simulink model "ver1_3DOF_draft2"  (R2023b)
settings: Solver=FixedStepAuto  StartTime=5  StopTime=45  RelTol=1e-3
values from neighbouring files (symbols this model uses):
  current_height = 0.0    (= 0)    [wrapper_for_simulink.m]
  current_pitch = 0.0    (= 0)    [wrapper_for_simulink.m]
  current_vel = 0.0    (= 0)    [wrapper_for_simulink.m]
  extension_length = 0.0    (= 0)    [wrapper_for_simulink.m]
undefined symbols (not defined in the file or in its folder): HDBK, Light, magnitude, MIL
libraries: aerolibwind2 x3, aerolibasang x2, aerolibadyn x1, aerolibatmos2 x1
settings Model: Creator=User  LastModifiedBy=User
settings DataIOCC: ReturnWorkspaceOutputsName=tp3ca22a37_fc90_43f8_8ebe_8c0e39ad763e
settings DebuggingCC: AlgebraicLoopMsg=none  ArtificialAlgebraicLoopMsg=none  ModelReferenceExtraNoncontSigs=none  OperatingPointInterfaceChecksumMismatchMsg=none

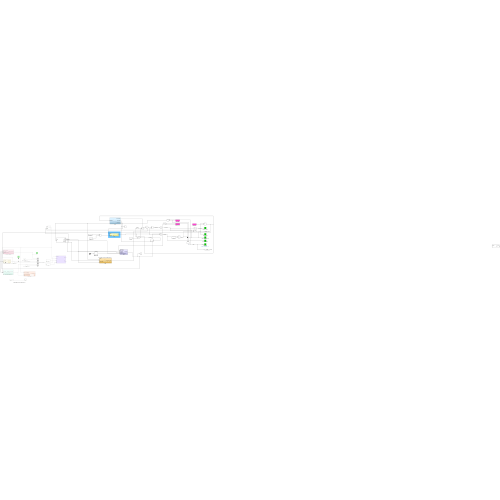
[thumbnail: Simulink's stored preview of the top-level diagram]
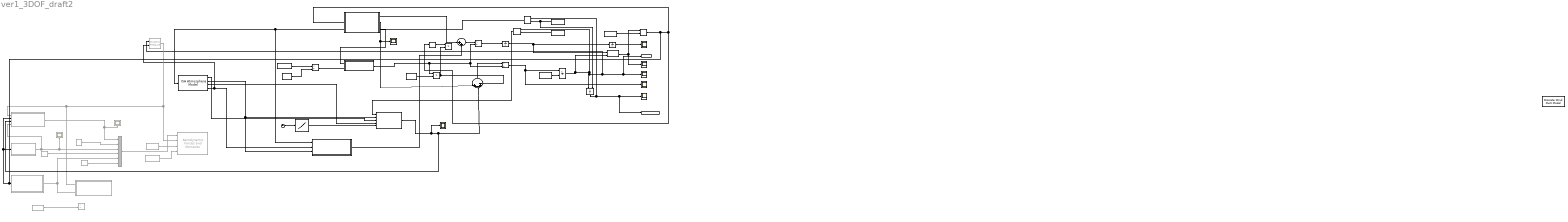
== system ver1_3DOF_draft2 ==
  note: ignore everything after v = 0
  note: need to figure out how the wind parameters here
  note: pitch damping moment: see pg 44 of OR doc
  " m(t)" : Subsystem
  "Aerodynamic Forces and Moments " : aerolibadyn/Aerodynamic Forces and Moments   Commented=on  inputAxes=Body  outputForceAxes=Body  outputMomentAxes=Body  S=0.016513  b=2.91  cbar=0.145
  Atan2 : Trigonometry  Operator=atan2
  Axial force coefficient : Subsystem  Commented=on
  CG rocket : Constant  Commented=on  Value=[0 0 1.16]  VectorParams1D=off
  CP rocket : Constant  Commented=on  Value=[0 0 0.95]  VectorParams1D=off
  Clock : Clock
  Delay1 : Delay  DelayLength=1  InitialConditionSource=Input port
      settings: InputPortMap=u0,p4
  Delay2 : Delay  DelayLength=1  InitialConditionSource=Input port
      settings: InputPortMap=u0,p4
  Delay3 : Delay  DelayLength=1  InitialConditionSource=Input port
      settings: InputPortMap=u0,p4
  Discrete Wind Gust Model : aerolibwind2/Discrete Wind Gust Model  units=Metric (MKS)  Gx=on  Gy=on  Gz=on  t_0=5  d_m=[120 120 80]  v_m=[3.5 3.5 3.0]
  Divide : Product  Inputs=*/
  Divide1 : Product  Inputs=*/
  Divide2 : Product  Inputs=*/
  Divide3 : Product  Commented=on  Inputs=*/
  Dynamic Pressure : aerolibasang/Dynamic Pressure  Commented=on
  Extension Plan : Lookup_n-D  NumberOfTableDimensions=1  BreakpointsForDimension1=[0 4.99 5 5.1 5.11 6]  Table=[0 0 extension_length 0.01*extension_length 0 0]  InternalRulePriority=Speed  RndMeth=Simplest
  Flight path angle : Scope
  ISA Atmosphere Model : aerolibatmos2/ISA Atmosphere Model  useExtended=off  action=Warning  custom=on  viscosityOut=off  g=9.80665  gamma=1.4  R=287.0531  L=0.0065  h_trop=11000  h_strat=20000  rho0=1.002  P0=86503.88  T0=temperature  h0=1401
  Integrator : Integrator  InitialConditionSource=external
  Integrator1 : Integrator  InitialConditionSource=external
  Integrator2 : Integrator
  Integrator3 : Integrator
  Normal Force coefficient : Subsystem  Commented=on
  Pitch moment : Subsystem  Commented=on
  Pitch moment coefficient : Subsystem  Commented=on
  Product1 : Product
  Product2 : Product
  Scope : Scope
  Scope1 : Scope  Commented=on
  Scope2 : Scope
  Scope4 : Scope  Commented=on
  Side force coefficient : Constant  Commented=on  Value=0
  Sin : Trigonometry
  Sum : Sum  Inputs=|+--+-
  Sum1 : Sum  Inputs=|++
  Vector Concatenate : Concatenate  Commented=on  NumInputs=6
  WIND : Subsystem
  current height : Constant  Value=current_height
  current pitch : Constant  Value=current_pitch
  current vel : Constant  Value=current_vel
  current velocity : Constant  Value=current_vel
  drag : Subsystem
  gravity g : Constant  Value=9.80665
  horizontal distance : Scope
  moi : Constant  Commented=on  Value=18.065
  propellant mass : Constant  Value=10.048
  roll moment coefficient : Constant  Commented=on  Value=0
  thrust : Subsystem
  total impulse : Constant  Value=21384.0
  vertical acceleration : Scope
  vertical height : Scope
  vertical velocity in earth ref : Scope
  yaw moment coefficient : Constant  Commented=on  Value=0
  Out1 : Outport  SignalName=height
  Out2 : Outport  Port=2  SignalName=velocity
  wires:
  Integrator1/1 -> Atan2/2, Integrator/1, Dynamic Pressure/1, Out2/1, vertical velocity in earth ref/1, Delay2/1  "velocity"
  ISA Atmosphere Model/2 -> WIND/3(speed of sound), drag/2(speed of sound)  "speed of sound"
  Sum/1 -> Divide1/1
  thrust/2(vertical thrust) -> Scope/1, Sum/1
  Delay2/1 -> drag/1(velocity vector)
  current velocity/1 -> Delay2/2
  current pitch/1 -> Delay1/2
  ISA Atmosphere Model/4 -> Dynamic Pressure/2, WIND/2(In2)
  " m(t)"/1(m(t)) -> Product1/1, Divide1/2, Divide2/2
  thrust/3(magnitude of T) -> " m(t)"/1(thrust)
  Integrator/1 -> Delay3/1, Out1/1, vertical height/1  "height"
  gravity g/1 -> Product1/2
  total impulse/1 -> Divide/1
  propellant mass/1 -> Divide/2
  Divide/1 -> " m(t)"/2(exhaust velocity)
  Divide1/1 -> Integrator1/1, vertical acceleration/1  "vertical accel"
  Atan2/1 -> Delay1/1, Flight path angle/1
  Delay3/1 -> ISA Atmosphere Model/1, WIND/1(Altitude)
  Sum1/1 -> Divide2/1  "Fx"
  WIND/1(wind force u direction) -> Sum1/2
  Integrator2/1 -> Atan2/1, Integrator3/1  "horizontal vel"
  Divide2/1 -> Integrator2/1  "horizontal accel"
  Product1/1 -> Sum/5, Product2/2  "gravitational"
  Sin/1 -> Product2/1
  thrust/1(horizontal thrust) -> Sum1/1
  Clock/1 -> Extension Plan/1
  current vel/1 -> Integrator1/2
  current height/1 -> Delay3/2, Integrator/2
  ISA Atmosphere Model/3 -> drag/4(pressure(Pa))
  Extension Plan/1 -> drag/5(Airbrakes extension plan)
  CG rocket/1 -> "Aerodynamic Forces and Moments "/3
  Vector Concatenate/1 -> "Aerodynamic Forces and Moments "/1  "aerodynamic coefficients"
  yaw moment coefficient/1 -> Vector Concatenate/6
  Pitch moment coefficient/1(pitch moment coefficient) -> Pitch moment/2(pitch moment coefficient), Vector Concatenate/5
  Normal Force coefficient/1(Normal) -> Axial force coefficient/4(Normal Force coefficient), Vector Concatenate/3, Scope1/1  "Normal Force coefficient"
  moi/1 -> Divide3/2
  Side force coefficient/1 -> Vector Concatenate/2
  Dynamic Pressure/1 -> "Aerodynamic Forces and Moments "/2, Pitch moment/1(dynammic pressure), Axial force coefficient/1(dynammic pressure)
  Delay1/1 -> Axial force coefficient/2(pitch angle), Normal Force coefficient/1(pitch angle), Pitch moment coefficient/1(pitch angle), Sin/1, thrust/1(pitch angle)
  CP rocket/1 -> "Aerodynamic Forces and Moments "/4
  Axial force coefficient/1("axial force coefficient ") -> Scope4/1, Vector Concatenate/1
  drag/1(Drag Force) -> Scope2/1, Axial force coefficient/3(Drag Force), Sum/3
  roll moment coefficient/1 -> Vector Concatenate/4
  Integrator3/1 -> horizontal distance/1  "horizontal dist"
  ISA Atmosphere Model/1 -> drag/3(temperature)

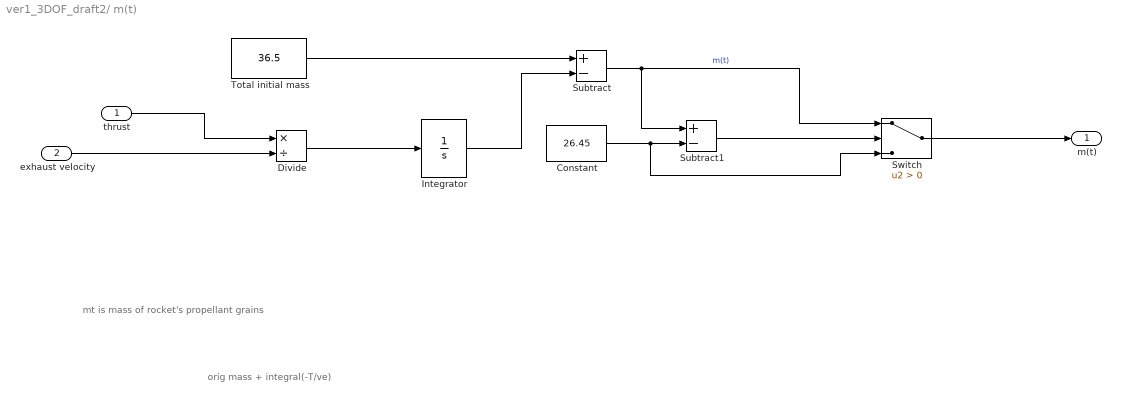
== system ver1_3DOF_draft2/ m(t) ==
  note: orig mass + integral(-T/ve)
  note: mt is mass of rocket's propellant grains
  thrust : Inport
  exhaust velocity : Inport  Port=2
  Constant : Constant  Value=26.45
  Divide : Product  Inputs=*/
  Integrator : Integrator
  Subtract : Sum  Inputs=+-
  Subtract1 : Sum  Inputs=+-
  Switch : Switch  Criteria=u2 > Threshold  SaturateOnIntegerOverflow=off  InputSameDT=off
  Total initial mass : Constant  Value=36.5
  m(t) : Outport
  wires:
  Total initial mass/1 -> Subtract/1
  Subtract/1 -> Subtract1/1, Switch/1  "m(t)"
  thrust/1 -> Divide/1
  exhaust velocity/1 -> Divide/2
  Divide/1 -> Integrator/1
  Integrator/1 -> Subtract/2
  Switch/1 -> m(t)/1
  Constant/1 -> Switch/3, Subtract1/2
  Subtract1/1 -> Switch/2

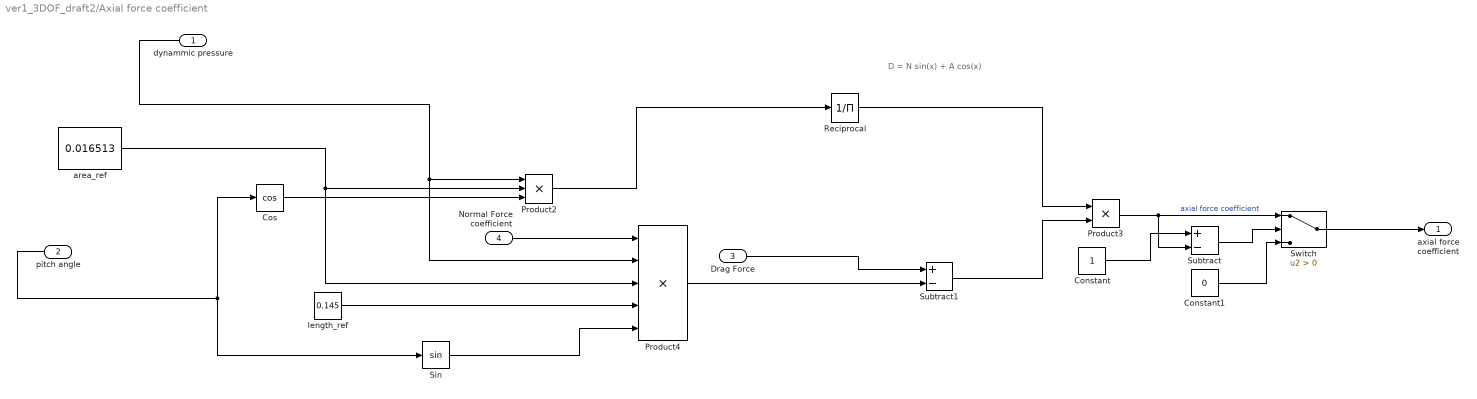
== system ver1_3DOF_draft2/Axial force coefficient ==
  note: D = N sin(x) + A cos(x)
  dynammic pressure : Inport
  pitch angle : Inport  Port=2
  Drag Force : Inport  Port=3
  Normal Force coefficient : Inport  Port=4
  Constant : Constant
  Constant1 : Constant  Value=0
  Cos : Trigonometry  Operator=cos
  Product2 : Product  Inputs=3
  Product3 : Product
  Product4 : Product  Inputs=5
  Reciprocal : Product  Inputs=/
  Sin : Trigonometry
  Subtract : Sum  Inputs=+-
  Subtract1 : Sum  Inputs=+-
  Switch : Switch  Criteria=u2 > Threshold  SaturateOnIntegerOverflow=off  InputSameDT=off
  area_ref : Constant  Value=0.016513
  length_ref : Constant  Value=0.145
  "axial force coefficient " : Outport
  wires:
  Sin/1 -> Product4/5
  pitch angle/1 -> Sin/1, Cos/1
  Normal Force coefficient/1 -> Product4/1
  dynammic pressure/1 -> Product4/2, Product2/1
  area_ref/1 -> Product2/2, Product4/3
  Cos/1 -> Product2/3
  length_ref/1 -> Product4/4
  Product4/1 -> Subtract1/2
  Product3/1 -> Subtract/2, Switch/1  "axial force coefficient"
  Subtract1/1 -> Product3/2
  Drag Force/1 -> Subtract1/1
  Product2/1 -> Reciprocal/1
  Reciprocal/1 -> Product3/1
  Switch/1 -> "axial force coefficient "/1
  Constant/1 -> Subtract/1
  Subtract/1 -> Switch/2
  Constant1/1 -> Switch/3

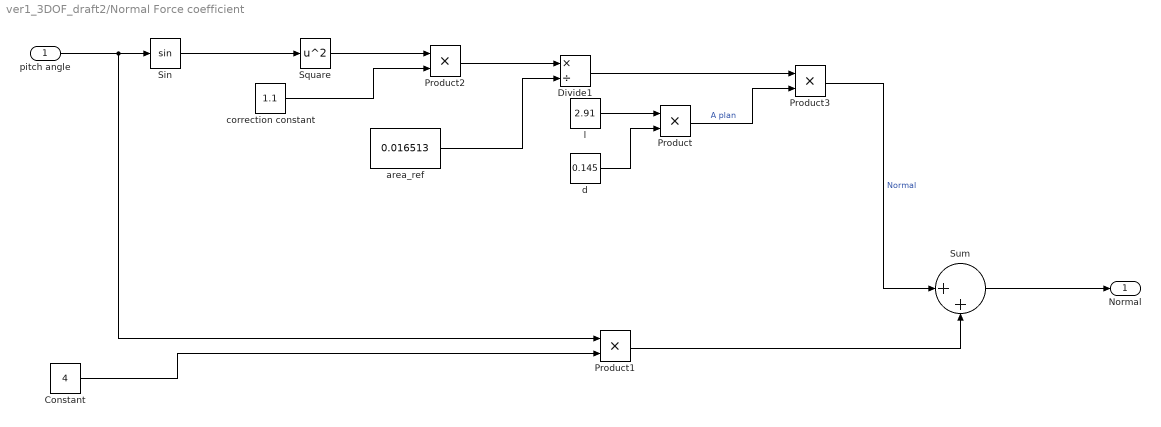
== system ver1_3DOF_draft2/Normal Force coefficient ==
  pitch angle : Inport
  Constant : Constant  Value=4
  Divide1 : Product  Inputs=*/
  Product{,1..3} (4 alike) : Product
  Sin : Trigonometry
  Square : Math  Operator=square
  Sum : Sum  Inputs=|++
  area_ref : Constant  Value=0.016513
  correction constant : Constant  Value=1.1
  d : Constant  Value=0.145
  l : Constant  Value=2.91
  Normal : Outport
  wires:
  pitch angle/1 -> Product1/1, Sin/1
  correction constant/1 -> Product2/2
  Product2/1 -> Divide1/1
  area_ref/1 -> Divide1/2
  Divide1/1 -> Product3/1
  Sin/1 -> Square/1
  Square/1 -> Product2/1
  Product/1 -> Product3/2  "A plan"
  l/1 -> Product/1
  d/1 -> Product/2
  Constant/1 -> Product1/2
  Product1/1 -> Sum/2
  Product3/1 -> Sum/1  "Normal"
  Sum/1 -> Normal/1

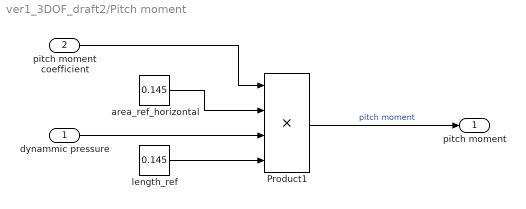
== system ver1_3DOF_draft2/Pitch moment ==
  dynammic pressure : Inport
  pitch moment coefficient : Inport  Port=2
  Product1 : Product  Inputs=4
  area_ref_horizontal : Constant  Value=0.145
  length_ref : Constant  Value=0.145
  pitch moment : Outport
  wires:
  area_ref_horizontal/1 -> Product1/2
  Product1/1 -> pitch moment/1  "pitch moment"
  length_ref/1 -> Product1/4
  dynammic pressure/1 -> Product1/3
  pitch moment coefficient/1 -> Product1/1

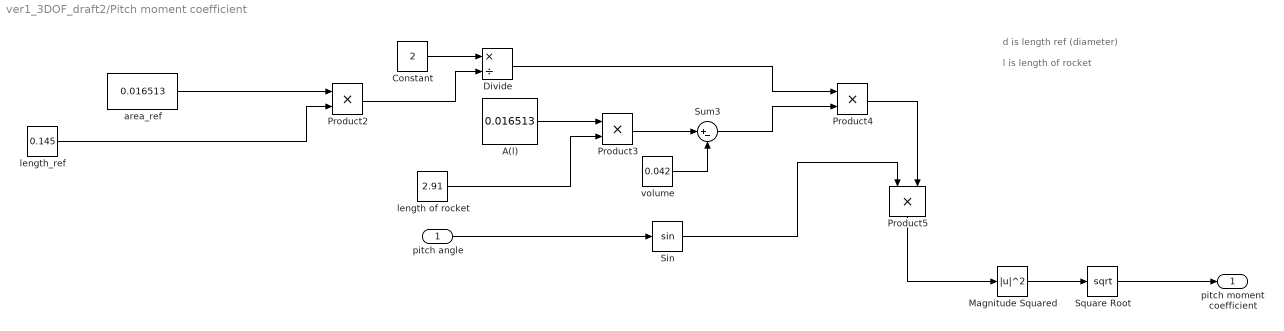
== system ver1_3DOF_draft2/Pitch moment coefficient ==
  note: l is length of rocket
  note: d is length ref (diameter)
  pitch angle : Inport
  A(l) : Constant  Value=0.016513
  Constant : Constant  Value=2
  Divide : Product  Inputs=*/
  Magnitude Squared : Math  Operator=magnitude^2
  Product{2..5} (4 alike) : Product
  Sin : Trigonometry
  Square Root : Sqrt
  Sum3 : Sum  Inputs=|+-
  area_ref : Constant  Value=0.016513
  length of rocket : Constant  Value=2.91
  length_ref : Constant  Value=0.145
  volume : Constant  Value=0.042
  pitch moment coefficient : Outport
  wires:
  length_ref/1 -> Product2/2
  Product2/1 -> Divide/2
  A(l)/1 -> Product3/1
  Product4/1 -> Product5/2
  Product5/1 -> Magnitude Squared/1
  area_ref/1 -> Product2/1
  Product3/1 -> Sum3/1
  Divide/1 -> Product4/1
  volume/1 -> Sum3/2
  Constant/1 -> Divide/1
  pitch angle/1 -> Sin/1
  Sum3/1 -> Product4/2
  Sin/1 -> Product5/1
  length of rocket/1 -> Product3/2
  Magnitude Squared/1 -> Square Root/1
  Square Root/1 -> pitch moment coefficient/1

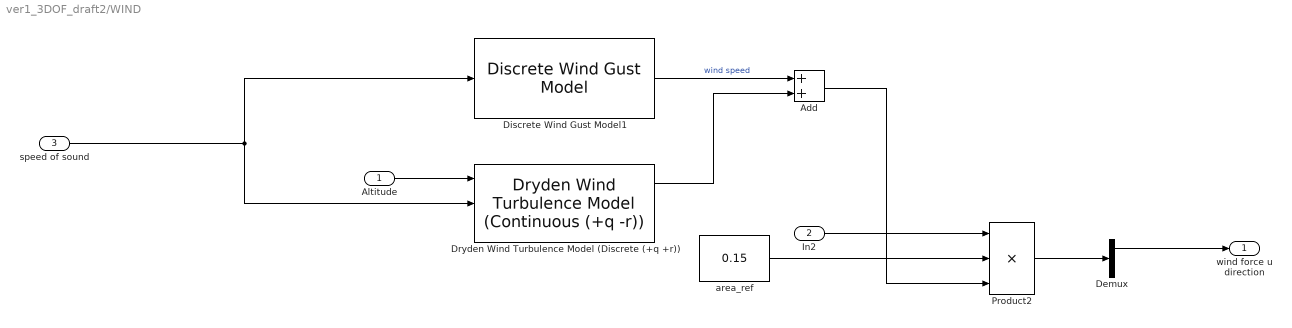
== system ver1_3DOF_draft2/WIND ==
  Altitude : Inport
  In2 : Inport  Port=2
  speed of sound : Inport  Port=3
  Add : Sum
  Demux : Demux  Outputs=3
  Discrete Wind Gust Model1 : aerolibwind2/Discrete Wind Gust Model  units=Metric (MKS)  Gx=on  Gy=on  Gz=on  t_0=0  d_m=[1 1 1]  v_m=[0 0 0]
  Dryden Wind Turbulence Model (Discrete (+q +r)) : aerolibwind2/Dryden Wind Turbulence Model  (Continuous (+q -r))  units=Metric (MKS)  spec=MIL-HDBK-1797B  model=Discrete Dryden (+q +r)  W20=0  Wdeg=4  TurbProb=10^-2 - Light  L_high=533.4  Wingspan=10  ts=0.1  Seed=[23341 23342 23343 23344]  T_on=on
      settings: LibrarySourceBlock=|
      | aerolibwind2/Dryden Wind Turbulence Model
      | (Discrete (+q +r))
  Product2 : Product  Inputs=3
  area_ref : Constant  Value=0.15
  wind force u direction : Outport
  wires:
  In2/1 -> Product2/1
  area_ref/1 -> Product2/2
  Dryden Wind Turbulence Model (Discrete (+q +r))/1 -> Add/2
  speed of sound/1 -> Discrete Wind Gust Model1/1, Dryden Wind Turbulence Model (Discrete (+q +r))/2
  Product2/1 -> Demux/1
  Altitude/1 -> Dryden Wind Turbulence Model (Discrete (+q +r))/1
  Discrete Wind Gust Model1/1 -> Add/1  "wind speed"
  Add/1 -> Product2/3
  Demux/1 -> wind force u direction/1

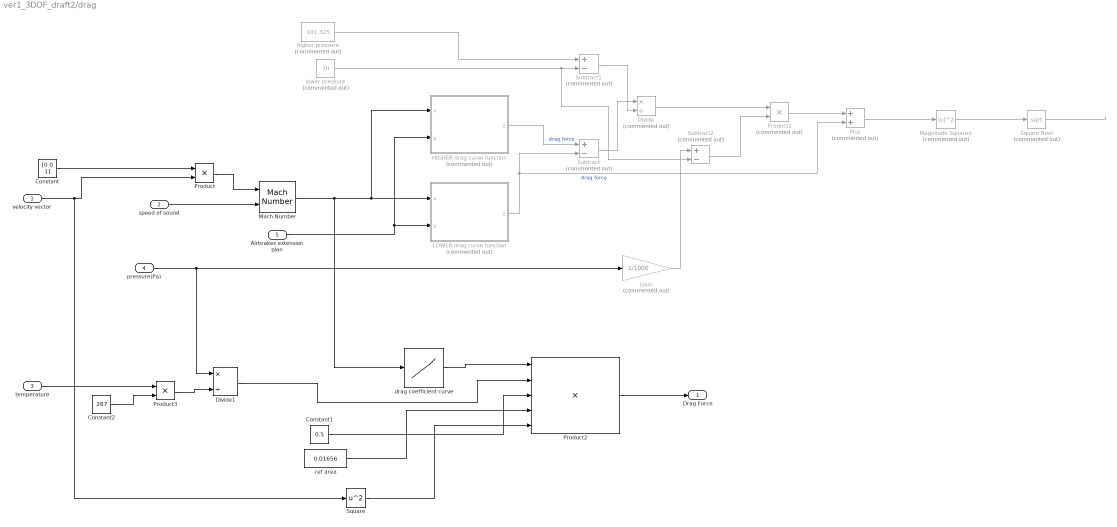
== system ver1_3DOF_draft2/drag ==
  velocity vector : Inport
  speed of sound : Inport  Port=2
  temperature : Inport  Port=3
  pressure(Pa) : Inport  Port=4
  Airbrakes extension plan : Inport  Port=5
  Constant : Constant  Value=[0 0 1]  VectorParams1D=off
  Constant1 : Constant  Value=0.5
  Constant2 : Constant  Value=287
  Divide : Product  Commented=on  Inputs=*/
  Divide1 : Product  Inputs=*/
  Gain : Gain  Commented=on  Gain=1/1000
  HIGHER drag curve function : MATLAB Function  Commented=on  TreatAsAtomicUnit=on
  LOWER drag curve function : MATLAB Function  Commented=on  TreatAsAtomicUnit=on
  Mach Number : aerolibasang/Mach Number
  Magnitude Squared : Math  Commented=on  Operator=magnitude^2
  Plus : Sum  Commented=on
  Product : Product
  Product1 : Product  Commented=on
  Product2 : Product  Inputs=5
  Product3 : Product
  Square : Math  Operator=square
  Square Root : Sqrt  Commented=on
  Subtract : Sum  Commented=on  Inputs=+-
  Subtract1 : Sum  Commented=on  Inputs=+-
  Subtract2 : Sum  Commented=on  Inputs=+-
  drag coefficient curve : Lookup_n-D  NumberOfTableDimensions=1  BreakpointsForDimension1=|  Table=|  InternalRulePriority=Speed  RndMeth=Simplest
      BreakpointsForDimension1=|
      | [0.025
      | 0.075
      | 0.125
      | 0.175
      | 0.225
      | 0.275
      | 0.3
      | 0.325
      | 0.35
      | 0.375
      | 0.4
      | 0.425
      | 0.45
      | 0.475
      | 0.5
      | 0.525
      | 0.55
      | 0.575
      | 0.6
      | 0.625
      | 0.65
      | 0.675
      | 0.7
      | 0.725
      | 0.75
      | 0.775
      | 0.8
      | 0.825
      | 0.85
      | 0.875
      | 0.9
      | 0.925
      | 0.95
      | 0.96
      | 0.97
      | 0.975
      | 0.98
      | 0.99
      | 1
      | 1.025
      | 1.03
      | 1.04
      | 1.05
      | 1.08
      | 1.09
      | 1.1
      | 1.11
      | 1.12
      | 1.125
      | 1.13
      | 1.14
      | 1.15
      | 1.16
      | 1.17
      | 1.175
      | 1.18
      | 1.19
      | 1.2
      | 1.25
      | 1.3
      | 1.35
      | 1.4
      | 1.45
      | 1.5
      | 1.55
      | 1.6
      | 1.65
      | 1.7
      | 1.75
      | 1.8
      | 1.85
      | 1.9
      | 1.95
      | 2]
      Table=|
      | [0.414355663
      | 0.348220023
      | 0.323436783
      | 0.308737589
      | 0.298518822
      | 0.290762121
      | 0.284796701
      | 0.281981595
      | 0.279419873
      | 0.277057421
      | 0.274906231
      | 0.272939302
      | 0.271147678
      | 0.269517368
      | 0.268043125
      | 0.266723372
      | 0.265624717
      | 0.264581106
      | 0.263628356
      | 0.262844663
      | 0.262127003
      | 0.261573935
      | 0.261178859
      | 0.260947896
      | 0.260908395
      | 0.261155796
      | 0.261965072
      | 0.264123632
      | 0.269418388
      | 0.279409465
      | 0.292628254
      | 0.304847858
      | 0.386158911
      | 0.418892417
      | 0.442585754
      | 0.460029047
      | 0.474019522
      | 0.521942821
      | 0.540871829
      | 0.55851086
      | 0.566684884
      | 0.566516984
      | 0.568307827
      | 0.552985866
      | 0.546166287
      | 0.539569504
      | 0.542370877
      | 0.539027596
      | 0.543481923
      | 0.535947193
      | 0.534214763
      | 0.530455789
      | 0.530231681
      | 0.527017666
      | 0.524954444
      | 0.523832601
      | 0.521303112
      | 0.519922467
      | 0.509373215
      | 0.498551065
      | 0.487444076
      | 0.477822288
      | 0.46864366
      | 0.459678358
      | 0.451228835
      | 0.443070568
      | 0.435650056
      | 0.42877815
      | 0.422263555
      | 0.416103972
      | 0.410274249
      | 0.404688363
      | 0.399198362
      | 0.393738487]
  higher pressure : Constant  Commented=on  Value=101.325
  lower pressure : Constant  Commented=on  Value=70
  ref area : Constant  Value=0.01656
  Drag Force : Outport
  wires:
  Mach Number/1 -> drag coefficient curve/1, HIGHER drag curve function/1(x), LOWER drag curve function/1(x)
  speed of sound/1 -> Mach Number/2
  Constant/1 -> Product/1
  Product/1 -> Mach Number/1
  Magnitude Squared/1 -> Square Root/1
  Square Root/1 -> ?
  Airbrakes extension plan/1 -> HIGHER drag curve function/2(y), LOWER drag curve function/2(y)
  HIGHER drag curve function/1(z) -> Subtract/1  "drag force"
  LOWER drag curve function/1(z) -> Plus/2, Subtract/2  "drag force"
  lower pressure/1 -> Subtract2/2, Subtract1/2
  higher pressure/1 -> Subtract1/1
  Subtract/1 -> Divide/1
  Subtract1/1 -> Divide/2
  Divide/1 -> Product1/1
  pressure(Pa)/1 -> Divide1/1, Gain/1
  Gain/1 -> Subtract2/1
  Subtract2/1 -> Product1/2
  Product1/1 -> Plus/1
  Plus/1 -> Magnitude Squared/1
  drag coefficient curve/1 -> Product2/1
  Divide1/1 -> Product2/2
  Constant1/1 -> Product2/3
  Product2/1 -> Drag Force/1
  ref area/1 -> Product2/4
  velocity vector/1 -> Square/1, Product/2
  Square/1 -> Product2/5
  temperature/1 -> Product3/1
  Constant2/1 -> Product3/2
  Product3/1 -> Divide1/2

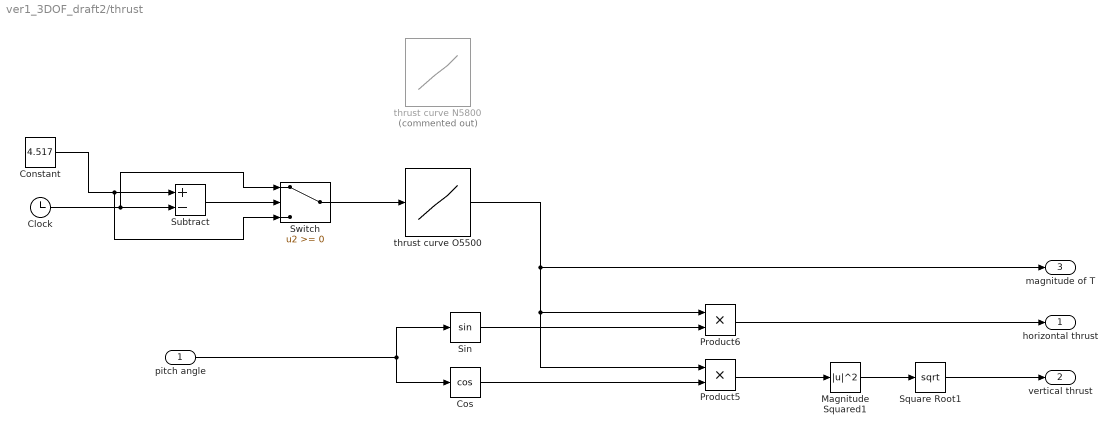
== system ver1_3DOF_draft2/thrust ==
  pitch angle : Inport
  Clock : Clock
  Constant : Constant  Value=4.517
  Cos : Trigonometry  Operator=cos
  Magnitude Squared1 : Math  Operator=magnitude^2
  Product5 : Product
  Product6 : Product
  Sin : Trigonometry
  Square Root1 : Sqrt
  Subtract : Sum  Inputs=+-
  Switch : Switch  SaturateOnIntegerOverflow=off  InputSameDT=off
  thrust curve N5800 : Lookup_n-D  Commented=on  NumberOfTableDimensions=1  BreakpointsForDimension1=|  BreakpointsForDimension2=[1:3]  Table=|  InternalRulePriority=Speed  RndMeth=Simplest
      BreakpointsForDimension1=|
      | [0.019
      | 0.049
      | 0.103
      | 0.384
      | 1.109
      | 1.569
      | 1.991
      | 2.622
      | 3.011
      | 3.192
      | 3.334
      | 3.423
      | 3.513
      | 3.581
      | 3.594]
      Table=|
      | [6694.9
      | 6720.292
      | 6593.334
      | 6677.973
      | 6957.279
      | 6940.352
      | 6720.292
      | 6009.329
      | 3275.507
      | 2606.864
      | 1599.666
      | 1041.053
      | 389.337
      | 220.06
      | 0.0]
  thrust curve O5500 : Lookup_n-D  NumberOfTableDimensions=1  BreakpointsForDimension1=|  BreakpointsForDimension2=[1:3]  Table=|  InternalRulePriority=Speed  RndMeth=Simplest
      BreakpointsForDimension1=|
      | [0.02
      | 0.063
      | 0.116
      | 0.206
      | 0.349
      | 0.578
      | 0.921
      | 1.378
      | 1.834
      | 2.29
      | 2.746
      | 2.87
      | 3.202
      | 3.659
      | 3.999
      | 4.19
      | 4.38
      | 4.487
      | 4.517]
      Table=|
      | [97.51531498
      | 5878.535832
      | 6146.986029
      | 6321
      | 6313.794354
      | 6286.771406
      | 6281.544745
      | 6265.531146
      | 6213.598154
      | 6137.533558
      | 6164.890123
      | 6079
      | 4268.057057
      | 2843.958783
      | 1793.95598
      | 1242.265247
      | 513.7576886
      | 77.83193263
      | 0]
  horizontal thrust : Outport
  vertical thrust : Outport  Port=2
  magnitude of T : Outport  Port=3
  wires:
  Clock/1 -> Switch/1, Subtract/2
  thrust curve O5500/1 -> Product6/1, Product5/1, magnitude of T/1
  Cos/1 -> Product5/2
  Sin/1 -> Product6/2
  pitch angle/1 -> Sin/1, Cos/1
  Product5/1 -> Magnitude Squared1/1
  Subtract/1 -> Switch/2
  Constant/1 -> Switch/3, Subtract/1
  Switch/1 -> thrust curve O5500/1
  Product6/1 -> horizontal thrust/1
  Magnitude Squared1/1 -> Square Root1/1
  Square Root1/1 -> vertical thrust/1

== matlab function ver1_3DOF_draft2/drag/LOWER drag curve function ==
  data: x input; z output; y input
function z = fcn(x, y)
%x is mach number, y is extension in m
z = 15.9894 - 81.7799 * x -1.7041e+03 *y + 280.5132*x^2 + 6.2419e+03*x*y + 2.7922e+04*y^2;

== matlab function ver1_3DOF_draft2/drag/HIGHER drag curve function ==
  data: x input; z output; y input
function z = fcn(x, y)
%x is mach number, y is extension in m
z = 23.6982 -123.4344*x - 2.5545e+03*y + 402.1042*x^2 + 9.1165e+03*x*y + 4.4646e+04*y^2;
